simulink model "EnergyMonitor_ThreePhase"  (R2022b)
settings: Solver=ode45  StartTime=0.0  StopTime=0.1  MaxStep=1e-5  RelTol=1e-3
model workspace (MAT data in the model file):
  R1 = 995.4722
  R2 = 663.648133333
  R3 = 497.7361
  Vpeak_1ph = 325.269119346
  Vpeak_3ph = 315.511045765
  Vrms_1ph = 230
  Vrms_3ph = 223.1
  XL = 2
  eta_xfmr = 0.97
  freq = 50
  omega = 314.159265359
  phi_A = 0
  phi_B = -2.09439510239
  phi_C = 2.09439510239
settings Model: Creator=User  LastModifiedBy=User

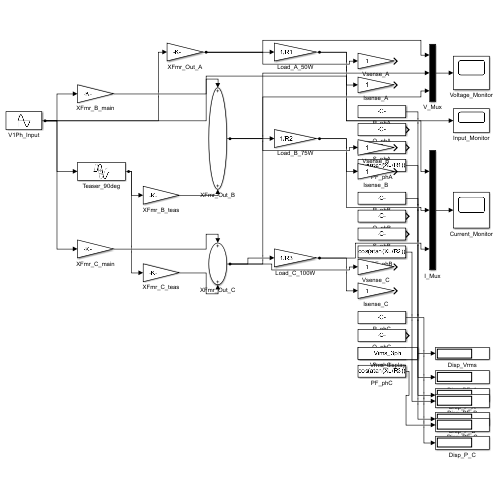
[thumbnail: Simulink's stored preview of the top-level diagram]
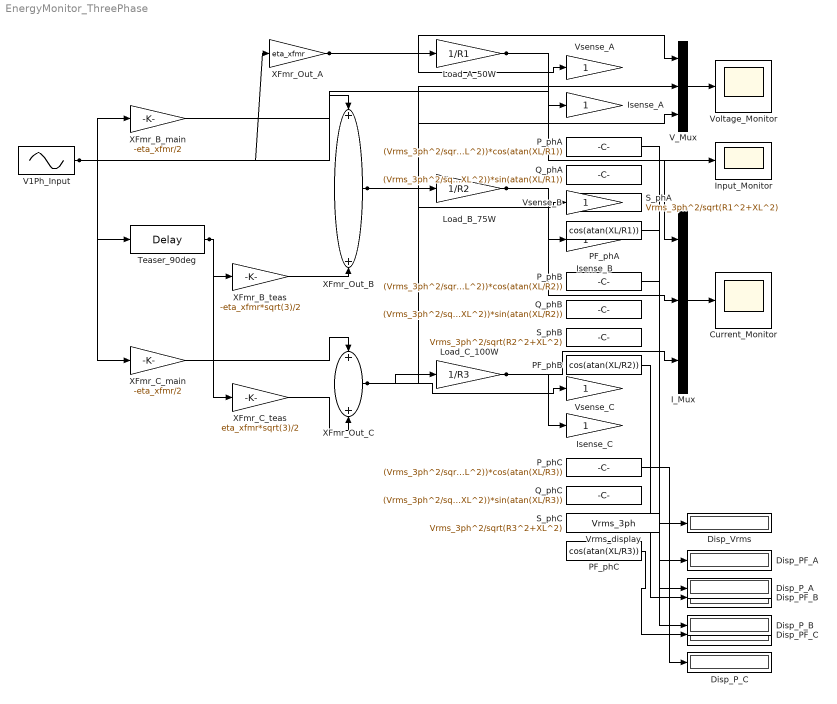
== system EnergyMonitor_ThreePhase ==
  Current_Monitor : Scope
  Disp_PF_A : Display
  Disp_PF_B : Display
  Disp_PF_C : Display
  Disp_P_A : Display
  Disp_P_B : Display
  Disp_P_C : Display
  Disp_Vrms : Display
  I_Mux : Mux  Inputs=3
  Input_Monitor : Scope
  Isense_A : Gain
  Isense_B : Gain
  Isense_C : Gain
  Load_A_50W : Gain  Gain=1/R1
  Load_B_75W : Gain  Gain=1/R2
  Load_C_100W : Gain  Gain=1/R3
  PF_phA : Constant  Value=cos(atan(XL/R1))
  PF_phB : Constant  Value=cos(atan(XL/R2))
  PF_phC : Constant  Value=cos(atan(XL/R3))
  P_phA : Constant  Value=(Vrms_3ph^2/sqrt(R1^2+XL^2))*cos(atan(XL/R1))
  P_phB : Constant  Value=(Vrms_3ph^2/sqrt(R2^2+XL^2))*cos(atan(XL/R2))
  P_phC : Constant  Value=(Vrms_3ph^2/sqrt(R3^2+XL^2))*cos(atan(XL/R3))
  Q_phA : Constant  Value=(Vrms_3ph^2/sqrt(R1^2+XL^2))*sin(atan(XL/R1))
  Q_phB : Constant  Value=(Vrms_3ph^2/sqrt(R2^2+XL^2))*sin(atan(XL/R2))
  Q_phC : Constant  Value=(Vrms_3ph^2/sqrt(R3^2+XL^2))*sin(atan(XL/R3))
  S_phA : Constant  Value=Vrms_3ph^2/sqrt(R1^2+XL^2)
  S_phB : Constant  Value=Vrms_3ph^2/sqrt(R2^2+XL^2)
  S_phC : Constant  Value=Vrms_3ph^2/sqrt(R3^2+XL^2)
  Teaser_90deg : TransportDelay  DelayTime=1/(4*freq)
  V1Ph_Input : Sin  Amplitude=Vpeak_1ph  Frequency=omega  SampleTime=0
  V_Mux : Mux  Inputs=3
  Voltage_Monitor : Scope
  Vrms_display : Constant  Value=Vrms_3ph
  Vsense_A : Gain
  Vsense_B : Gain
  Vsense_C : Gain
  XFmr_B_main : Gain  Gain=-eta_xfmr/2
  XFmr_B_teas : Gain  Gain=-eta_xfmr*sqrt(3)/2
  XFmr_C_main : Gain  Gain=-eta_xfmr/2
  XFmr_C_teas : Gain  Gain=eta_xfmr*sqrt(3)/2
  XFmr_Out_A : Gain  Gain=eta_xfmr
  XFmr_Out_B : Sum
  XFmr_Out_C : Sum
  wires:
  V1Ph_Input/1 -> Teaser_90deg/1, XFmr_Out_A/1, XFmr_B_main/1, XFmr_C_main/1, Input_Monitor/1
  Teaser_90deg/1 -> XFmr_B_teas/1, XFmr_C_teas/1
  XFmr_B_main/1 -> XFmr_Out_B/1
  XFmr_B_teas/1 -> XFmr_Out_B/2
  XFmr_C_main/1 -> XFmr_Out_C/1
  XFmr_C_teas/1 -> XFmr_Out_C/2
  XFmr_Out_A/1 -> Load_A_50W/1, Vsense_A/1, V_Mux/1
  XFmr_Out_B/1 -> Load_B_75W/1, Vsense_B/1, V_Mux/2
  XFmr_Out_C/1 -> Load_C_100W/1, Vsense_C/1, V_Mux/3
  Load_A_50W/1 -> Isense_A/1, I_Mux/1
  Load_B_75W/1 -> Isense_B/1, I_Mux/2
  Load_C_100W/1 -> Isense_C/1, I_Mux/3
  V_Mux/1 -> Voltage_Monitor/1
  I_Mux/1 -> Current_Monitor/1
  PF_phA/1 -> Disp_PF_A/1
  P_phA/1 -> Disp_P_A/1
  PF_phB/1 -> Disp_PF_B/1
  P_phB/1 -> Disp_P_B/1
  PF_phC/1 -> Disp_PF_C/1
  P_phC/1 -> Disp_P_C/1
  Vrms_display/1 -> Disp_Vrms/1
